simulink model "ATRIAS_anim_static_floor"  (R2014b)
settings: Solver=ode45  StartTime=0.0  StopTime=sim_t  FixedStep=1e-3  RelTol=1e-3  AbsTol=1e-4
undefined symbols (not defined in the file): base_color_d, boom_color_d, d_com, fblink_color_d, floor_color_d, floor_tile_width, floor_zero_height, g, hshaft_color_d, l_seg, lowerleg_12, lowerleg_color_d, m_boom, m_fblink, m_hshaft, m_lowerleg, m_output_gear, m_rotor, m_shin, m_thigh, m_torso, m_total, m_virtual_gear, m_yshaft, r_hip_gearhead, r_hip_shaft, r_rotor, r_virtual_gear, shin_12, shin_color_d, shin_initial_l, shin_initial_r, thigh_color_d, thigh_initial_l, thigh_initial_r, tile_color, tile_cross_section, tile_delta, tile_scale_visual, torso_color_d, X, Y, yshaft_color_d, Z
libraries: sm_lib x186, nesl_utility x85
(part 3 of 5)

== system ATRIAS_anim_static_floor/ATRIAS Mechanics Layer/ATRIAS Mechanical System Layer/L Hip Shaft/Frame Data ==
  Mux : Mux  Inputs=3
  PS-Simulink Converter{,1..3} (4 alike) : nesl_utility/PS-Simulink Converter  PhysicalDomain=network_engine_domain  SubClassName=ps_output  LeftPortType=input  RightPortType=output  PseudoPeriodic=off  Frequencies=[]  Unit=1  AffineConversion=off
  Transform Sensor : sm_lib/Frames and Transforms/Transform Sensor  MeasurementFrame=World  SenseAngle=off  SenseAxis=off  SenseAngle1=off  SenseAngle2=off  SenseAngle3=off  SenseQ=on  SenseR=off  SenseOmegaX=off  SenseOmegaY=off  SenseOmegaZ=off  SenseOmega1=off  SenseOmega2=off  SenseOmega3=off  SenseQDot=off  SenseRDot=off  SenseAlphaX=off  SenseAlphaY=off  SenseAlphaZ=off  SenseAlpha1=off  SenseAlpha2=off  SenseAlpha3=off  SenseQDDot=off  SenseRDDot=off  SenseX=on  SenseY=on  SenseZ=on  SenseRad=off  SenseAzim=off  SenseDist=off  SenseInc=off  SenseXDot=off  SenseYDot=off  SenseZDot=off  SenseRadDot=off  SenseAzimDot=off  SenseDistDot=off  SenseIncDot=off  SenseXDDot=off  SenseYDDot=off  SenseZDDot=off  SenseRadDDot=off  SenseAzimDDot=off  SenseDistDDot=off  SenseIncDDot=off  BlockFunction=simmechanics.library.frames_transforms.transform_sensor
  World Frame : sm_lib/Frames and Transforms/World Frame  BlockFunction=simmechanics.library.frames_transforms.world_frame
  Frame : PMIOPort  Port=1  Side=Left
  tag scope: LQHipShaft=global, LxyzHipShaft=global
  wires:
  PS-Simulink Converter/1 -> [LQHipShaft]
  PS-Simulink Converter1/1 -> Mux/1
  PS-Simulink Converter2/1 -> Mux/2
  PS-Simulink Converter3/1 -> Mux/3
  Mux/1 -> [LxyzHipShaft]
  connections:
  Transform Sensor/RConn1 -- Frame/RConn1
  Transform Sensor/LConn1 -- World Frame/RConn1
  Transform Sensor/RConn2 -- PS-Simulink Converter/LConn1
  Transform Sensor/RConn5 -- PS-Simulink Converter3/LConn1
  Transform Sensor/RConn3 -- PS-Simulink Converter1/LConn1
  Transform Sensor/RConn4 -- PS-Simulink Converter2/LConn1

== system ATRIAS_anim_static_floor/ATRIAS Mechanics Layer/ATRIAS Mechanical System Layer/L Leg/Angle Range Map1 ==
  "[0,2*pi]" : Inport
  Constant1 : Constant  Value=pi
  Constant2 : Constant  Value=pi
  Sum1 : Sum  Inputs=-+|
  Sum2 : Sum  Inputs=|+-
  Switch1 : Switch  ZeroCross=off
  "[-pi,pi]" : Outport
  wires:
  "[0,2*pi]"/1 -> Switch1/3, Sum1/2, Sum2/1
  Switch1/1 -> "[-pi,pi]"/1
  Constant2/1 -> Sum2/2
  Sum2/1 -> Switch1/2
  Sum1/1 -> Switch1/1
  Constant1/1 -> Sum1/1

== system ATRIAS_anim_static_floor/ATRIAS Mechanics Layer/ATRIAS Mechanical System Layer/L Leg/Angle Range Map2 ==
  "[0,2*pi]" : Inport
  Constant1 : Constant  Value=pi
  Constant2 : Constant  Value=pi
  Sum1 : Sum  Inputs=-+|
  Sum2 : Sum  Inputs=|+-
  Switch1 : Switch  ZeroCross=off
  "[-pi,pi]" : Outport
  wires:
  "[0,2*pi]"/1 -> Switch1/3, Sum1/2, Sum2/1
  Switch1/1 -> "[-pi,pi]"/1
  Constant2/1 -> Sum2/2
  Sum2/1 -> Switch1/2
  Sum1/1 -> Switch1/1
  Constant1/1 -> Sum1/1

== system ATRIAS_anim_static_floor/ATRIAS Mechanics Layer/ATRIAS Mechanical System Layer/L Leg/Four Bar Link ==
  CS1 to CS2 : sm_lib/Frames and Transforms/Rigid Transform  TranslationMethod=Cartesian  TranslationLengthUnit=m  TranslationStandardAxis=+Z  TranslationStandardOffset=0  TranslationCartesianOffset=[0 -l_seg 0]  TranslationROffset=0  TranslationROffsetUnits=m  TranslationZOffset=0  TranslationZOffsetUnits=m  TranslationThetaOffset=0  TranslationThetaOffsetUnits=deg  RotationMethod=None  RotationAngleUnits=deg  RotationStandardAxis=+Z  RotationAngle=0  RotationArbitraryAxis=[0 0 1]  FollAlignAxisA=+X  BaseAlignAxisA=+Y  FollAlignAxisB=+Y  BaseAlignAxisB=+Z  RotationMatrix=[1 0 0; 0 1 0; 0 0 1]  BlockFunction=simmechanics.library.frames_transforms.rigid_transform
  Frame Data : Subsystem
  Solid : sm_lib/Body Elements/Solid  InertiaType=Custom  Mass=m_fblink  MassUnits=kg  CenterOfMass=com_fblink  CenterOfMassUnits=m  MomentsOfInertia=i_fblink_moments  MomentsOfInertiaUnits=kg*m^2  ProductsOfInertia=i_fblink_products  ProductsOfInertiaUnits=kg*m^2  DensityBased=on  Density=1000  DensityUnits=kg/(m^3)  GraphicType=FromGeometry  MarkerShape=Sphere  MarkerSize=10  MarkerSizeUnits=m  GraphicVisPropType=AdvancedVisualProperties  GraphicDiffuseColor=fblink_color_d  GraphicSpecularColor=[0.5 0.5 0.5 1.0]  GraphicAmbientColor=[fblink_color_d*0.5 1.0]  GraphicEmissiveColor=[0.0 0.0 0.0 1.0]  GraphicShininess=128  GraphicOpacity=1.0  GeometryShape=FromFile  RectangleSize=[1 1]  RectangleSizeUnits=m  BrickDimensions=[0.1 l_seg 0.1]  BrickDimensionUnits=m  CylinderRadius=l_rad  CylinderRadiusUnits=m  CylinderLength=l_seg  CylinderLengthUnits=m  SphereRadius=1  SphereRadiusUnits=m  EllipsoidRadii=[1 1 1]  EllipsoidRadiiUnits=m  ExtrusionCrossSection=[1 1; -1 1; -1 -1; 1 -1]  ExtrusionCrossSectionUnits=m  ExtrusionLength=1  ExtrusionLengthUnits=m  PolygonNumSides=3  PolygonOuterRadius=1  PolygonOuterRadiusUnits=m  ExtGeomFileType=STL  ExtGeomFileName=../0_images/models/four_bar_link.stl  ExtGeomFileUnits=m  RevolutionCrossSection=[1 1; 1 -1; 2 -1; 2 1]  RevolutionCrossSectionUnits=m  RevolutionExtent=Full  RevolutionAngle=180  RevolutionAngleUnits=deg  BlockFunction=simmechanics.library.body_elements.solid
  CS1 : PMIOPort  Port=1  Side=Left
  CS2 : PMIOPort  Port=2  Side=Right
  connections:
  CS2/RConn1 -- CS1 to CS2/RConn1
  Solid/RConn1 -- CS1/RConn1 -- Frame Data/LConn1 -- CS1 to CS2/LConn1

== system ATRIAS_anim_static_floor/ATRIAS Mechanics Layer/ATRIAS Mechanical System Layer/L Leg/Lower Leg ==
  CS1 to CS2 : sm_lib/Frames and Transforms/Rigid Transform  TranslationMethod=Cartesian  TranslationLengthUnit=m  TranslationStandardAxis=+Z  TranslationStandardOffset=0  TranslationCartesianOffset=[0 -lowerleg_12 0]  TranslationROffset=0  TranslationROffsetUnits=m  TranslationZOffset=0  TranslationZOffsetUnits=m  TranslationThetaOffset=0  TranslationThetaOffsetUnits=deg  RotationMethod=None  RotationAngleUnits=deg  RotationStandardAxis=+Z  RotationAngle=0  RotationArbitraryAxis=[0 0 1]  FollAlignAxisA=+X  BaseAlignAxisA=+Y  FollAlignAxisB=+Y  BaseAlignAxisB=+Z  RotationMatrix=[1 0 0; 0 1 0; 0 0 1]  BlockFunction=simmechanics.library.frames_transforms.rigid_transform
  CS1 to CS3 : sm_lib/Frames and Transforms/Rigid Transform  TranslationMethod=Cartesian  TranslationLengthUnit=m  TranslationStandardAxis=+Z  TranslationStandardOffset=0  TranslationCartesianOffset=[0 -l_seg 0]  TranslationROffset=0  TranslationROffsetUnits=m  TranslationZOffset=0  TranslationZOffsetUnits=m  TranslationThetaOffset=0  TranslationThetaOffsetUnits=deg  RotationMethod=None  RotationAngleUnits=deg  RotationStandardAxis=+Z  RotationAngle=0  RotationArbitraryAxis=[0 0 1]  FollAlignAxisA=+X  BaseAlignAxisA=+Y  FollAlignAxisB=+Y  BaseAlignAxisB=+Z  RotationMatrix=[1 0 0; 0 1 0; 0 0 1]  BlockFunction=simmechanics.library.frames_transforms.rigid_transform
  Frame Data : Subsystem
  Solid : sm_lib/Body Elements/Solid  InertiaType=Custom  Mass=m_lowerleg  MassUnits=kg  CenterOfMass=com_lowerleg  CenterOfMassUnits=m  MomentsOfInertia=i_lowerleg_moments  MomentsOfInertiaUnits=kg*m^2  ProductsOfInertia=i_lowerleg_products  ProductsOfInertiaUnits=kg*m^2  DensityBased=on  Density=1000  DensityUnits=kg/(m^3)  GraphicType=FromGeometry  MarkerShape=Sphere  MarkerSize=10  MarkerSizeUnits=m  GraphicVisPropType=AdvancedVisualProperties  GraphicDiffuseColor=lowerleg_color_d  GraphicSpecularColor=[0.5 0.5 0.5 1.0]  GraphicAmbientColor=[lowerleg_color_d*0.5 1.0]  GraphicEmissiveColor=[0.0 0.0 0.0 1.0]  GraphicShininess=128  GraphicOpacity=1.0  GeometryShape=FromFile  RectangleSize=[1 1]  RectangleSizeUnits=m  BrickDimensions=[0.1 l_seg 0.1]  BrickDimensionUnits=m  CylinderRadius=l_rad  CylinderRadiusUnits=m  CylinderLength=l_seg  CylinderLengthUnits=m  SphereRadius=1  SphereRadiusUnits=m  EllipsoidRadii=[1 1 1]  EllipsoidRadiiUnits=m  ExtrusionCrossSection=[1 1; -1 1; -1 -1; 1 -1]  ExtrusionCrossSectionUnits=m  ExtrusionLength=1  ExtrusionLengthUnits=m  PolygonNumSides=3  PolygonOuterRadius=1  PolygonOuterRadiusUnits=m  ExtGeomFileType=STL  ExtGeomFileName=../0_images/models/lower_leg.STL  ExtGeomFileUnits=m  RevolutionCrossSection=[1 1; 1 -1; 2 -1; 2 1]  RevolutionCrossSectionUnits=m  RevolutionExtent=Full  RevolutionAngle=180  RevolutionAngleUnits=deg  BlockFunction=simmechanics.library.body_elements.solid
  CS1 : PMIOPort  Port=1  Side=Left
  CS2 : PMIOPort  Port=2  Side=Right
  CS3 : PMIOPort  Port=3  Side=Right
  connections:
  CS3/RConn1 -- CS1 to CS3/RConn1
  Frame Data/LConn1 -- CS1 to CS3/LConn1 -- CS1 to CS2/LConn1 -- Solid/RConn1 -- CS1/RConn1
  CS2/RConn1 -- CS1 to CS2/RConn1

== system ATRIAS_anim_static_floor/ATRIAS Mechanics Layer/ATRIAS Mechanical System Layer/L Leg/Shin ==
  CS1 to CS2 : sm_lib/Frames and Transforms/Rigid Transform  TranslationMethod=Cartesian  TranslationLengthUnit=m  TranslationStandardAxis=+Z  TranslationStandardOffset=0  TranslationCartesianOffset=[0 -shin_12 0]  TranslationROffset=0  TranslationROffsetUnits=m  TranslationZOffset=0  TranslationZOffsetUnits=m  TranslationThetaOffset=0  TranslationThetaOffsetUnits=deg  RotationMethod=None  RotationAngleUnits=deg  RotationStandardAxis=+Z  RotationAngle=0  RotationArbitraryAxis=[0 0 1]  FollAlignAxisA=+X  BaseAlignAxisA=+Y  FollAlignAxisB=+Y  BaseAlignAxisB=+Z  RotationMatrix=[1 0 0; 0 1 0; 0 0 1]  BlockFunction=simmechanics.library.frames_transforms.rigid_transform
  Frame Data : Subsystem
  Solid : sm_lib/Body Elements/Solid  InertiaType=Custom  Mass=m_shin  MassUnits=kg  CenterOfMass=com_shin  CenterOfMassUnits=m  MomentsOfInertia=i_shin_moments  MomentsOfInertiaUnits=kg*m^2  ProductsOfInertia=i_shin_products  ProductsOfInertiaUnits=kg*m^2  DensityBased=on  Density=1000  DensityUnits=kg/(m^3)  GraphicType=FromGeometry  MarkerShape=Sphere  MarkerSize=10  MarkerSizeUnits=m  GraphicVisPropType=AdvancedVisualProperties  GraphicDiffuseColor=shin_color_d  GraphicSpecularColor=[0.5 0.5 0.5 1.0]  GraphicAmbientColor=[shin_color_d*0.5 1.0]  GraphicEmissiveColor=[0.0 0.0 0.0 1.0]  GraphicShininess=128  GraphicOpacity=1.0  GeometryShape=FromFile  RectangleSize=[1 1]  RectangleSizeUnits=m  BrickDimensions=[1 1 1]  BrickDimensionUnits=m  CylinderRadius=l_rad  CylinderRadiusUnits=m  CylinderLength=l_seg  CylinderLengthUnits=m  SphereRadius=1  SphereRadiusUnits=m  EllipsoidRadii=[1 1 1]  EllipsoidRadiiUnits=m  ExtrusionCrossSection=[1 1; -1 1; -1 -1; 1 -1]  ExtrusionCrossSectionUnits=m  ExtrusionLength=1  ExtrusionLengthUnits=m  PolygonNumSides=3  PolygonOuterRadius=1  PolygonOuterRadiusUnits=m  ExtGeomFileType=STL  ExtGeomFileName=../0_images/models/shin.STL  ExtGeomFileUnits=m  RevolutionCrossSection=[1 1; 1 -1; 2 -1; 2 1]  RevolutionCrossSectionUnits=m  RevolutionExtent=Full  RevolutionAngle=180  RevolutionAngleUnits=deg  BlockFunction=simmechanics.library.body_elements.solid
  CS1 : PMIOPort  Port=1  Side=Left
  CS2 : PMIOPort  Port=2  Side=Right
  connections:
  CS1 to CS2/LConn1 -- CS1/RConn1 -- Frame Data/LConn1 -- Solid/RConn1
  CS2/RConn1 -- CS1 to CS2/RConn1

== system ATRIAS_anim_static_floor/ATRIAS Mechanics Layer/ATRIAS Mechanical System Layer/L Leg/Shin SEA ==
  note: Shin SEA Mechanics
  Shin Gear [rad] : Inport
  Initial Gear Angle1 : Constant  Value=shin_initial_l
  Rotor and Gearing : Subsystem
  Sum1 : Sum  Inputs=-+|
  Terminator : Terminator
  Terminator1 : Terminator
  Rotor Joint Conn : PMIOPort  Port=1  Side=Left
  wires:
  Rotor and Gearing/2(Gearhead Velocity [rad/s]) -> Terminator/1
  Sum1/1 -> Rotor and Gearing/1(Shin Gear pos [rad])
  Shin Gear [rad]/1 -> Sum1/2
  Initial Gear Angle1/1 -> Sum1/1
  Rotor and Gearing/1(Gearhead Position [rad]) -> Terminator1/1
  connections:
  Rotor and Gearing/LConn1 -- Rotor Joint Conn/RConn1

== system ATRIAS_anim_static_floor/ATRIAS Mechanics Layer/ATRIAS Mechanical System Layer/L Leg/Thigh ==
  CS1 to CS2 : sm_lib/Frames and Transforms/Rigid Transform  TranslationMethod=Cartesian  TranslationLengthUnit=m  TranslationStandardAxis=+Z  TranslationStandardOffset=0  TranslationCartesianOffset=[0 -l_seg 0]  TranslationROffset=0  TranslationROffsetUnits=m  TranslationZOffset=0  TranslationZOffsetUnits=m  TranslationThetaOffset=0  TranslationThetaOffsetUnits=deg  RotationMethod=None  RotationAngleUnits=deg  RotationStandardAxis=+Z  RotationAngle=0  RotationArbitraryAxis=[0 0 1]  FollAlignAxisA=+X  BaseAlignAxisA=+Y  FollAlignAxisB=+Y  BaseAlignAxisB=+Z  RotationMatrix=[1 0 0; 0 1 0; 0 0 1]  BlockFunction=simmechanics.library.frames_transforms.rigid_transform
  Frame Data : Subsystem
  Solid : sm_lib/Body Elements/Solid  InertiaType=Custom  Mass=m_thigh  MassUnits=kg  CenterOfMass=com_thigh  CenterOfMassUnits=m  MomentsOfInertia=i_thigh_moments  MomentsOfInertiaUnits=kg*m^2  ProductsOfInertia=i_thigh_products  ProductsOfInertiaUnits=kg*m^2  DensityBased=on  Density=1000  DensityUnits=kg/(m^3)  GraphicType=FromGeometry  MarkerShape=Sphere  MarkerSize=10  MarkerSizeUnits=m  GraphicVisPropType=AdvancedVisualProperties  GraphicDiffuseColor=thigh_color_d  GraphicSpecularColor=[0.5 0.5 0.5 1.0]  GraphicAmbientColor=[thigh_color_d*0.5 1.0]  GraphicEmissiveColor=[0.0 0.0 0.0 1.0]  GraphicShininess=128  GraphicOpacity=1.0  GeometryShape=FromFile  RectangleSize=[1 1]  RectangleSizeUnits=m  BrickDimensions=[1 1 1]  BrickDimensionUnits=m  CylinderRadius=l_rad  CylinderRadiusUnits=m  CylinderLength=l_seg  CylinderLengthUnits=m  SphereRadius=1  SphereRadiusUnits=m  EllipsoidRadii=[1 1 1]  EllipsoidRadiiUnits=m  ExtrusionCrossSection=[1 1; -1 1; -1 -1; 1 -1]  ExtrusionCrossSectionUnits=m  ExtrusionLength=1  ExtrusionLengthUnits=m  PolygonNumSides=3  PolygonOuterRadius=1  PolygonOuterRadiusUnits=m  ExtGeomFileType=STL  ExtGeomFileName=../0_images/models/thigh.STL  ExtGeomFileUnits=m  RevolutionCrossSection=[1 1; 1 -1; 2 -1; 2 1]  RevolutionCrossSectionUnits=m  RevolutionExtent=Full  RevolutionAngle=180  RevolutionAngleUnits=deg  BlockFunction=simmechanics.library.body_elements.solid
  CS1 : PMIOPort  Port=1  Side=Left
  CS2 : PMIOPort  Port=2  Side=Right
  connections:
  CS2/RConn1 -- CS1 to CS2/RConn1
  CS1 to CS2/LConn1 -- Solid/RConn1 -- Frame Data/LConn1 -- CS1/RConn1

== system ATRIAS_anim_static_floor/ATRIAS Mechanics Layer/ATRIAS Mechanical System Layer/L Leg/Thigh SEA ==
  note: Thigh SEA Mechanics
  Thigh Gear [rad] : Inport
  Initial Gear Angle1 : Constant  Value=thigh_initial_l
  Rotor and Gearing : Subsystem
  Sum1 : Sum  Inputs=-+|
  Terminator : Terminator
  Terminator1 : Terminator
  Rotor Joint Conn : PMIOPort  Port=1  Side=Left
  wires:
  Rotor and Gearing/2(Gearhead Velocity [rad/s]) -> Terminator/1
  Sum1/1 -> Rotor and Gearing/1(Thigh Gear pos [rad])
  Initial Gear Angle1/1 -> Sum1/1
  Thigh Gear [rad]/1 -> Sum1/2
  Rotor and Gearing/1(Gearhead Position [rad]) -> Terminator1/1
  connections:
  Rotor and Gearing/LConn1 -- Rotor Joint Conn/RConn1

== system ATRIAS_anim_static_floor/ATRIAS Mechanics Layer/ATRIAS Mechanical System Layer/R Hip Shaft/Frame Data ==
  Mux : Mux  Inputs=3
  PS-Simulink Converter{,1..3} (4 alike) : nesl_utility/PS-Simulink Converter  PhysicalDomain=network_engine_domain  SubClassName=ps_output  LeftPortType=input  RightPortType=output  PseudoPeriodic=off  Frequencies=[]  Unit=1  AffineConversion=off
  Transform Sensor : sm_lib/Frames and Transforms/Transform Sensor  MeasurementFrame=World  SenseAngle=off  SenseAxis=off  SenseAngle1=off  SenseAngle2=off  SenseAngle3=off  SenseQ=on  SenseR=off  SenseOmegaX=off  SenseOmegaY=off  SenseOmegaZ=off  SenseOmega1=off  SenseOmega2=off  SenseOmega3=off  SenseQDot=off  SenseRDot=off  SenseAlphaX=off  SenseAlphaY=off  SenseAlphaZ=off  SenseAlpha1=off  SenseAlpha2=off  SenseAlpha3=off  SenseQDDot=off  SenseRDDot=off  SenseX=on  SenseY=on  SenseZ=on  SenseRad=off  SenseAzim=off  SenseDist=off  SenseInc=off  SenseXDot=off  SenseYDot=off  SenseZDot=off  SenseRadDot=off  SenseAzimDot=off  SenseDistDot=off  SenseIncDot=off  SenseXDDot=off  SenseYDDot=off  SenseZDDot=off  SenseRadDDot=off  SenseAzimDDot=off  SenseDistDDot=off  SenseIncDDot=off  BlockFunction=simmechanics.library.frames_transforms.transform_sensor
  World Frame : sm_lib/Frames and Transforms/World Frame  BlockFunction=simmechanics.library.frames_transforms.world_frame
  Frame : PMIOPort  Port=1  Side=Left
  tag scope: RQHipShaft=global, RxyzHipShaft=global
  wires:
  PS-Simulink Converter/1 -> [RQHipShaft]
  PS-Simulink Converter1/1 -> Mux/1
  PS-Simulink Converter2/1 -> Mux/2
  PS-Simulink Converter3/1 -> Mux/3
  Mux/1 -> [RxyzHipShaft]
  connections:
  Transform Sensor/RConn1 -- Frame/RConn1
  Transform Sensor/LConn1 -- World Frame/RConn1
  Transform Sensor/RConn3 -- PS-Simulink Converter1/LConn1
  Transform Sensor/RConn5 -- PS-Simulink Converter3/LConn1
  Transform Sensor/RConn4 -- PS-Simulink Converter2/LConn1
  Transform Sensor/RConn2 -- PS-Simulink Converter/LConn1

== system ATRIAS_anim_static_floor/ATRIAS Mechanics Layer/ATRIAS Mechanical System Layer/R Leg/Angle Range Map1 ==
  "[0,2*pi]" : Inport
  Constant1 : Constant  Value=pi
  Constant2 : Constant  Value=pi
  Sum1 : Sum  Inputs=-+|
  Sum2 : Sum  Inputs=|+-
  Switch1 : Switch  ZeroCross=off
  "[-pi,pi]" : Outport
  wires:
  "[0,2*pi]"/1 -> Switch1/3, Sum1/2, Sum2/1
  Switch1/1 -> "[-pi,pi]"/1
  Constant2/1 -> Sum2/2
  Sum2/1 -> Switch1/2
  Sum1/1 -> Switch1/1
  Constant1/1 -> Sum1/1

== system ATRIAS_anim_static_floor/ATRIAS Mechanics Layer/ATRIAS Mechanical System Layer/R Leg/Angle Range Map2 ==
  "[0,2*pi]" : Inport
  Constant1 : Constant  Value=pi
  Constant2 : Constant  Value=pi
  Sum1 : Sum  Inputs=-+|
  Sum2 : Sum  Inputs=|+-
  Switch1 : Switch  ZeroCross=off
  "[-pi,pi]" : Outport
  wires:
  "[0,2*pi]"/1 -> Switch1/3, Sum1/2, Sum2/1
  Switch1/1 -> "[-pi,pi]"/1
  Constant2/1 -> Sum2/2
  Sum2/1 -> Switch1/2
  Sum1/1 -> Switch1/1
  Constant1/1 -> Sum1/1

== system ATRIAS_anim_static_floor/ATRIAS Mechanics Layer/ATRIAS Mechanical System Layer/R Leg/Four Bar Link ==
  CS1 to CS2 : sm_lib/Frames and Transforms/Rigid Transform  TranslationMethod=Cartesian  TranslationLengthUnit=m  TranslationStandardAxis=+Z  TranslationStandardOffset=0  TranslationCartesianOffset=[0 -l_seg 0]  TranslationROffset=0  TranslationROffsetUnits=m  TranslationZOffset=0  TranslationZOffsetUnits=m  TranslationThetaOffset=0  TranslationThetaOffsetUnits=deg  RotationMethod=None  RotationAngleUnits=deg  RotationStandardAxis=+Z  RotationAngle=0  RotationArbitraryAxis=[0 0 1]  FollAlignAxisA=+X  BaseAlignAxisA=+Y  FollAlignAxisB=+Y  BaseAlignAxisB=+Z  RotationMatrix=[1 0 0; 0 1 0; 0 0 1]  BlockFunction=simmechanics.library.frames_transforms.rigid_transform
  Frame Data : Subsystem
  Solid : sm_lib/Body Elements/Solid  InertiaType=Custom  Mass=m_fblink  MassUnits=kg  CenterOfMass=com_fblink  CenterOfMassUnits=m  MomentsOfInertia=i_fblink_moments  MomentsOfInertiaUnits=kg*m^2  ProductsOfInertia=i_fblink_products  ProductsOfInertiaUnits=kg*m^2  DensityBased=on  Density=1000  DensityUnits=kg/(m^3)  GraphicType=FromGeometry  MarkerShape=Sphere  MarkerSize=10  MarkerSizeUnits=m  GraphicVisPropType=AdvancedVisualProperties  GraphicDiffuseColor=fblink_color_d  GraphicSpecularColor=[0.5 0.5 0.5 1.0]  GraphicAmbientColor=[fblink_color_d*0.5 1.0]  GraphicEmissiveColor=[0.0 0.0 0.0 1.0]  GraphicShininess=128  GraphicOpacity=1.0  GeometryShape=FromFile  RectangleSize=[1 1]  RectangleSizeUnits=m  BrickDimensions=[0.1 l_seg 0.1]  BrickDimensionUnits=m  CylinderRadius=l_rad  CylinderRadiusUnits=m  CylinderLength=l_seg  CylinderLengthUnits=m  SphereRadius=1  SphereRadiusUnits=m  EllipsoidRadii=[1 1 1]  EllipsoidRadiiUnits=m  ExtrusionCrossSection=[1 1; -1 1; -1 -1; 1 -1]  ExtrusionCrossSectionUnits=m  ExtrusionLength=1  ExtrusionLengthUnits=m  PolygonNumSides=3  PolygonOuterRadius=1  PolygonOuterRadiusUnits=m  ExtGeomFileType=STL  ExtGeomFileName=../0_images/models/four_bar_link.stl  ExtGeomFileUnits=m  RevolutionCrossSection=[1 1; 1 -1; 2 -1; 2 1]  RevolutionCrossSectionUnits=m  RevolutionExtent=Full  RevolutionAngle=180  RevolutionAngleUnits=deg  BlockFunction=simmechanics.library.body_elements.solid
  CS1 : PMIOPort  Port=1  Side=Left
  CS2 : PMIOPort  Port=2  Side=Right
  connections:
  CS2/RConn1 -- CS1 to CS2/RConn1
  Solid/RConn1 -- CS1/RConn1 -- Frame Data/LConn1 -- CS1 to CS2/LConn1

== system ATRIAS_anim_static_floor/ATRIAS Mechanics Layer/ATRIAS Mechanical System Layer/R Leg/Lower Leg ==
  CS1 to CS2 : sm_lib/Frames and Transforms/Rigid Transform  TranslationMethod=Cartesian  TranslationLengthUnit=m  TranslationStandardAxis=+Z  TranslationStandardOffset=0  TranslationCartesianOffset=[0 -lowerleg_12 0]  TranslationROffset=0  TranslationROffsetUnits=m  TranslationZOffset=0  TranslationZOffsetUnits=m  TranslationThetaOffset=0  TranslationThetaOffsetUnits=deg  RotationMethod=None  RotationAngleUnits=deg  RotationStandardAxis=+Z  RotationAngle=0  RotationArbitraryAxis=[0 0 1]  FollAlignAxisA=+X  BaseAlignAxisA=+Y  FollAlignAxisB=+Y  BaseAlignAxisB=+Z  RotationMatrix=[1 0 0; 0 1 0; 0 0 1]  BlockFunction=simmechanics.library.frames_transforms.rigid_transform
  CS1 to CS3 : sm_lib/Frames and Transforms/Rigid Transform  TranslationMethod=Cartesian  TranslationLengthUnit=m  TranslationStandardAxis=+Z  TranslationStandardOffset=0  TranslationCartesianOffset=[0 -l_seg 0]  TranslationROffset=0  TranslationROffsetUnits=m  TranslationZOffset=0  TranslationZOffsetUnits=m  TranslationThetaOffset=0  TranslationThetaOffsetUnits=deg  RotationMethod=None  RotationAngleUnits=deg  RotationStandardAxis=+Z  RotationAngle=0  RotationArbitraryAxis=[0 0 1]  FollAlignAxisA=+X  BaseAlignAxisA=+Y  FollAlignAxisB=+Y  BaseAlignAxisB=+Z  RotationMatrix=[1 0 0; 0 1 0; 0 0 1]  BlockFunction=simmechanics.library.frames_transforms.rigid_transform
  Frame Data : Subsystem
  Solid : sm_lib/Body Elements/Solid  InertiaType=Custom  Mass=m_lowerleg  MassUnits=kg  CenterOfMass=com_lowerleg  CenterOfMassUnits=m  MomentsOfInertia=i_lowerleg_moments  MomentsOfInertiaUnits=kg*m^2  ProductsOfInertia=i_lowerleg_products  ProductsOfInertiaUnits=kg*m^2  DensityBased=on  Density=1000  DensityUnits=kg/(m^3)  GraphicType=FromGeometry  MarkerShape=Sphere  MarkerSize=10  MarkerSizeUnits=m  GraphicVisPropType=AdvancedVisualProperties  GraphicDiffuseColor=lowerleg_color_d  GraphicSpecularColor=[0.5 0.5 0.5 1.0]  GraphicAmbientColor=[lowerleg_color_d*0.5 1.0]  GraphicEmissiveColor=[0.0 0.0 0.0 1.0]  GraphicShininess=128  GraphicOpacity=1.0  GeometryShape=FromFile  RectangleSize=[1 1]  RectangleSizeUnits=m  BrickDimensions=[0.1 l_seg 0.1]  BrickDimensionUnits=m  CylinderRadius=l_rad  CylinderRadiusUnits=m  CylinderLength=l_seg  CylinderLengthUnits=m  SphereRadius=1  SphereRadiusUnits=m  EllipsoidRadii=[1 1 1]  EllipsoidRadiiUnits=m  ExtrusionCrossSection=[1 1; -1 1; -1 -1; 1 -1]  ExtrusionCrossSectionUnits=m  ExtrusionLength=1  ExtrusionLengthUnits=m  PolygonNumSides=3  PolygonOuterRadius=1  PolygonOuterRadiusUnits=m  ExtGeomFileType=STL  ExtGeomFileName=../0_images/models/lower_leg.STL  ExtGeomFileUnits=m  RevolutionCrossSection=[1 1; 1 -1; 2 -1; 2 1]  RevolutionCrossSectionUnits=m  RevolutionExtent=Full  RevolutionAngle=180  RevolutionAngleUnits=deg  BlockFunction=simmechanics.library.body_elements.solid
  CS1 : PMIOPort  Port=1  Side=Left
  CS2 : PMIOPort  Port=2  Side=Right
  CS3 : PMIOPort  Port=3  Side=Right
  connections:
  CS3/RConn1 -- CS1 to CS3/RConn1
  CS1 to CS3/LConn1 -- CS1 to CS2/LConn1 -- Solid/RConn1 -- Frame Data/LConn1 -- CS1/RConn1
  CS2/RConn1 -- CS1 to CS2/RConn1

== system ATRIAS_anim_static_floor/ATRIAS Mechanics Layer/ATRIAS Mechanical System Layer/R Leg/Shin ==
  CS1 to CS2 : sm_lib/Frames and Transforms/Rigid Transform  TranslationMethod=Cartesian  TranslationLengthUnit=m  TranslationStandardAxis=+Z  TranslationStandardOffset=0  TranslationCartesianOffset=[0 -shin_12 0]  TranslationROffset=0  TranslationROffsetUnits=m  TranslationZOffset=0  TranslationZOffsetUnits=m  TranslationThetaOffset=0  TranslationThetaOffsetUnits=deg  RotationMethod=None  RotationAngleUnits=deg  RotationStandardAxis=+Z  RotationAngle=0  RotationArbitraryAxis=[0 0 1]  FollAlignAxisA=+X  BaseAlignAxisA=+Y  FollAlignAxisB=+Y  BaseAlignAxisB=+Z  RotationMatrix=[1 0 0; 0 1 0; 0 0 1]  BlockFunction=simmechanics.library.frames_transforms.rigid_transform
  Frame Data : Subsystem
  Solid : sm_lib/Body Elements/Solid  InertiaType=Custom  Mass=m_shin  MassUnits=kg  CenterOfMass=com_shin  CenterOfMassUnits=m  MomentsOfInertia=i_shin_moments  MomentsOfInertiaUnits=kg*m^2  ProductsOfInertia=i_shin_products  ProductsOfInertiaUnits=kg*m^2  DensityBased=on  Density=1000  DensityUnits=kg/(m^3)  GraphicType=FromGeometry  MarkerShape=Sphere  MarkerSize=10  MarkerSizeUnits=m  GraphicVisPropType=AdvancedVisualProperties  GraphicDiffuseColor=shin_color_d  GraphicSpecularColor=[0.5 0.5 0.5 1.0]  GraphicAmbientColor=[shin_color_d*0.5 1.0]  GraphicEmissiveColor=[0.0 0.0 0.0 1.0]  GraphicShininess=128  GraphicOpacity=1.0  GeometryShape=FromFile  RectangleSize=[1 1]  RectangleSizeUnits=m  BrickDimensions=[1 1 1]  BrickDimensionUnits=m  CylinderRadius=l_rad  CylinderRadiusUnits=m  CylinderLength=l_seg  CylinderLengthUnits=m  SphereRadius=1  SphereRadiusUnits=m  EllipsoidRadii=[1 1 1]  EllipsoidRadiiUnits=m  ExtrusionCrossSection=[1 1; -1 1; -1 -1; 1 -1]  ExtrusionCrossSectionUnits=m  ExtrusionLength=1  ExtrusionLengthUnits=m  PolygonNumSides=3  PolygonOuterRadius=1  PolygonOuterRadiusUnits=m  ExtGeomFileType=STL  ExtGeomFileName=../0_images/models/shin.STL  ExtGeomFileUnits=m  RevolutionCrossSection=[1 1; 1 -1; 2 -1; 2 1]  RevolutionCrossSectionUnits=m  RevolutionExtent=Full  RevolutionAngle=180  RevolutionAngleUnits=deg  BlockFunction=simmechanics.library.body_elements.solid
  CS1 : PMIOPort  Port=1  Side=Left
  CS2 : PMIOPort  Port=2  Side=Right
  connections:
  CS1 to CS2/LConn1 -- CS1/RConn1 -- Frame Data/LConn1 -- Solid/RConn1
  CS2/RConn1 -- CS1 to CS2/RConn1

== system ATRIAS_anim_static_floor/ATRIAS Mechanics Layer/ATRIAS Mechanical System Layer/R Leg/Shin SEA ==
  note: Shin SEA Mechanics
  Shin Gear Pos [rad] : Inport
  Initial Gear Angle1 : Constant  Value=shin_initial_r
  Rotor and Gearing : Subsystem
  Sum1 : Sum  Inputs=-+|
  Terminator : Terminator
  Terminator1 : Terminator
  Rotor Joint Conn : PMIOPort  Port=1  Side=Left
  wires:
  Sum1/1 -> Rotor and Gearing/1(Gear position [rad])
  Shin Gear Pos [rad]/1 -> Sum1/2
  Initial Gear Angle1/1 -> Sum1/1
  Rotor and Gearing/2(Gearhead Velocity [rad/s]) -> Terminator/1
  Rotor and Gearing/1(Gearhead Position [rad]) -> Terminator1/1
  connections:
  Rotor and Gearing/LConn1 -- Rotor Joint Conn/RConn1

== system ATRIAS_anim_static_floor/ATRIAS Mechanics Layer/ATRIAS Mechanical System Layer/R Leg/Thigh ==
  CS1 to CS2 : sm_lib/Frames and Transforms/Rigid Transform  TranslationMethod=Cartesian  TranslationLengthUnit=m  TranslationStandardAxis=+Z  TranslationStandardOffset=0  TranslationCartesianOffset=[0 -l_seg 0]  TranslationROffset=0  TranslationROffsetUnits=m  TranslationZOffset=0  TranslationZOffsetUnits=m  TranslationThetaOffset=0  TranslationThetaOffsetUnits=deg  RotationMethod=None  RotationAngleUnits=deg  RotationStandardAxis=+Z  RotationAngle=0  RotationArbitraryAxis=[0 0 1]  FollAlignAxisA=+X  BaseAlignAxisA=+Y  FollAlignAxisB=+Y  BaseAlignAxisB=+Z  RotationMatrix=[1 0 0; 0 1 0; 0 0 1]  BlockFunction=simmechanics.library.frames_transforms.rigid_transform
  Frame Data : Subsystem
  Solid : sm_lib/Body Elements/Solid  InertiaType=Custom  Mass=m_thigh  MassUnits=kg  CenterOfMass=com_thigh  CenterOfMassUnits=m  MomentsOfInertia=i_thigh_moments  MomentsOfInertiaUnits=kg*m^2  ProductsOfInertia=i_thigh_products  ProductsOfInertiaUnits=kg*m^2  DensityBased=on  Density=1000  DensityUnits=kg/(m^3)  GraphicType=FromGeometry  MarkerShape=Sphere  MarkerSize=10  MarkerSizeUnits=m  GraphicVisPropType=AdvancedVisualProperties  GraphicDiffuseColor=thigh_color_d  GraphicSpecularColor=[0.5 0.5 0.5 1.0]  GraphicAmbientColor=[thigh_color_d*0.5 1.0]  GraphicEmissiveColor=[0.0 0.0 0.0 1.0]  GraphicShininess=128  GraphicOpacity=1.0  GeometryShape=FromFile  RectangleSize=[1 1]  RectangleSizeUnits=m  BrickDimensions=[1 1 1]  BrickDimensionUnits=m  CylinderRadius=l_rad  CylinderRadiusUnits=m  CylinderLength=l_seg  CylinderLengthUnits=m  SphereRadius=1  SphereRadiusUnits=m  EllipsoidRadii=[1 1 1]  EllipsoidRadiiUnits=m  ExtrusionCrossSection=[1 1; -1 1; -1 -1; 1 -1]  ExtrusionCrossSectionUnits=m  ExtrusionLength=1  ExtrusionLengthUnits=m  PolygonNumSides=3  PolygonOuterRadius=1  PolygonOuterRadiusUnits=m  ExtGeomFileType=STL  ExtGeomFileName=../0_images/models/thigh.STL  ExtGeomFileUnits=m  RevolutionCrossSection=[1 1; 1 -1; 2 -1; 2 1]  RevolutionCrossSectionUnits=m  RevolutionExtent=Full  RevolutionAngle=180  RevolutionAngleUnits=deg  BlockFunction=simmechanics.library.body_elements.solid
  CS1 : PMIOPort  Port=1  Side=Left
  CS2 : PMIOPort  Port=2  Side=Right
  connections:
  CS2/RConn1 -- CS1 to CS2/RConn1
  CS1 to CS2/LConn1 -- Solid/RConn1 -- Frame Data/LConn1 -- CS1/RConn1

== system ATRIAS_anim_static_floor/ATRIAS Mechanics Layer/ATRIAS Mechanical System Layer/R Leg/Thigh SEA ==
  note: Thigh SEA Mechanics
  Thigh Gear [rad] : Inport
  Initial Gear Angle1 : Constant  Value=thigh_initial_r
  Rotor and Gearing : Subsystem
  Sum1 : Sum  Inputs=-+|
  Terminator : Terminator
  Terminator1 : Terminator
  Rotor Joint Conn : PMIOPort  Port=1  Side=Left
  wires:
  Sum1/1 -> Rotor and Gearing/1(Thigh Gear pos [rad])
  Initial Gear Angle1/1 -> Sum1/1
  Thigh Gear [rad]/1 -> Sum1/2
  Rotor and Gearing/2(Gearhead Velocity [rad/s]) -> Terminator/1
  Rotor and Gearing/1(Gearhead Position [rad]) -> Terminator1/1
  connections:
  Rotor and Gearing/LConn1 -- Rotor Joint Conn/RConn1

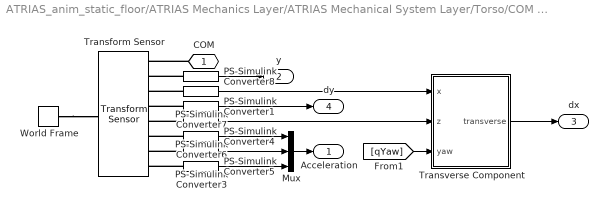
== system ATRIAS_anim_static_floor/ATRIAS Mechanics Layer/ATRIAS Mechanical System Layer/Torso/COM Sensor ==
  Mux : Mux  Inputs=3
  PS-Simulink Converter{1,3..8} (7 alike) : nesl_utility/PS-Simulink Converter  PhysicalDomain=network_engine_domain  SubClassName=ps_output  LeftPortType=input  RightPortType=output  PseudoPeriodic=off  Frequencies=[]  Unit=1  AffineConversion=off
  Transform Sensor : sm_lib/Frames and Transforms/Transform Sensor  MeasurementFrame=World  SenseAngle=off  SenseAxis=off  SenseAngle1=off  SenseAngle2=off  SenseAngle3=off  SenseQ=off  SenseR=off  SenseOmegaX=off  SenseOmegaY=off  SenseOmegaZ=off  SenseOmega1=off  SenseOmega2=off  SenseOmega3=off  SenseQDot=off  SenseRDot=off  SenseAlphaX=off  SenseAlphaY=off  SenseAlphaZ=off  SenseAlpha1=off  SenseAlpha2=off  SenseAlpha3=off  SenseQDDot=off  SenseRDDot=off  SenseX=off  SenseY=on  SenseZ=off  SenseRad=off  SenseAzim=off  SenseDist=off  SenseInc=off  SenseXDot=on  SenseYDot=on  SenseZDot=on  SenseRadDot=off  SenseAzimDot=off  SenseDistDot=off  SenseIncDot=off  SenseXDDot=on  SenseYDDot=on  SenseZDDot=on  SenseRadDDot=off  SenseAzimDDot=off  SenseDistDDot=off  SenseIncDDot=off  BlockFunction=simmechanics.library.frames_transforms.transform_sensor
  Transverse Component : Subsystem
  World Frame : sm_lib/Frames and Transforms/World Frame  BlockFunction=simmechanics.library.frames_transforms.world_frame
  COM : PMIOPort  Port=1  Side=Left
  Acceleration : Outport
  y : Outport  Port=2
  dx : Outport  Port=3
  dy : Outport  Port=4
  wires:
  PS-Simulink Converter5/1 -> Mux/3
  Mux/1 -> Acceleration/1
  PS-Simulink Converter8/1 -> y/1
  PS-Simulink Converter3/1 -> Mux/2
  PS-Simulink Converter4/1 -> Mux/1
  PS-Simulink Converter7/1 -> Transverse Component/1(x)
  Transverse Component/1(transverse) -> dx/1
  [qYaw] -> Transverse Component/3(yaw)
  PS-Simulink Converter1/1 -> dy/1
  PS-Simulink Converter6/1 -> Transverse Component/2(z)
  connections:
  COM/RConn1 -- Transform Sensor/RConn1
  World Frame/RConn1 -- Transform Sensor/LConn1
  PS-Simulink Converter5/LConn1 -- Transform Sensor/RConn8
  PS-Simulink Converter3/LConn1 -- Transform Sensor/RConn7
  PS-Simulink Converter4/LConn1 -- Transform Sensor/RConn6
  PS-Simulink Converter6/LConn1 -- Transform Sensor/RConn5
  PS-Simulink Converter7/LConn1 -- Transform Sensor/RConn3
  PS-Simulink Converter8/LConn1 -- Transform Sensor/RConn2
  PS-Simulink Converter1/LConn1 -- Transform Sensor/RConn4

== system ATRIAS_anim_static_floor/ATRIAS Mechanics Layer/ATRIAS Mechanical System Layer/Torso/Frame Data ==
  Mux : Mux  Inputs=3
  PS-Simulink Converter{,1..3} (4 alike) : nesl_utility/PS-Simulink Converter  PhysicalDomain=network_engine_domain  SubClassName=ps_output  LeftPortType=input  RightPortType=output  PseudoPeriodic=off  Frequencies=[]  Unit=1  AffineConversion=off
  Transform Sensor : sm_lib/Frames and Transforms/Transform Sensor  MeasurementFrame=World  SenseAngle=off  SenseAxis=off  SenseAngle1=off  SenseAngle2=off  SenseAngle3=off  SenseQ=on  SenseR=off  SenseOmegaX=off  SenseOmegaY=off  SenseOmegaZ=off  SenseOmega1=off  SenseOmega2=off  SenseOmega3=off  SenseQDot=off  SenseRDot=off  SenseAlphaX=off  SenseAlphaY=off  SenseAlphaZ=off  SenseAlpha1=off  SenseAlpha2=off  SenseAlpha3=off  SenseQDDot=off  SenseRDDot=off  SenseX=on  SenseY=on  SenseZ=on  SenseRad=off  SenseAzim=off  SenseDist=off  SenseInc=off  SenseXDot=off  SenseYDot=off  SenseZDot=off  SenseRadDot=off  SenseAzimDot=off  SenseDistDot=off  SenseIncDot=off  SenseXDDot=off  SenseYDDot=off  SenseZDDot=off  SenseRadDDot=off  SenseAzimDDot=off  SenseDistDDot=off  SenseIncDDot=off  BlockFunction=simmechanics.library.frames_transforms.transform_sensor
  World Frame : sm_lib/Frames and Transforms/World Frame  BlockFunction=simmechanics.library.frames_transforms.world_frame
  Frame : PMIOPort  Port=1  Side=Left
  tag scope: QTorso=global, xyzTorso=global
  wires:
  PS-Simulink Converter/1 -> [QTorso]
  PS-Simulink Converter1/1 -> Mux/1
  PS-Simulink Converter2/1 -> Mux/2
  PS-Simulink Converter3/1 -> Mux/3
  Mux/1 -> [xyzTorso]
  connections:
  Transform Sensor/RConn1 -- Frame/RConn1
  Transform Sensor/LConn1 -- World Frame/RConn1
  Transform Sensor/RConn5 -- PS-Simulink Converter3/LConn1
  Transform Sensor/RConn4 -- PS-Simulink Converter2/LConn1
  Transform Sensor/RConn3 -- PS-Simulink Converter1/LConn1
  Transform Sensor/RConn2 -- PS-Simulink Converter/LConn1

== system ATRIAS_anim_static_floor/ATRIAS Mechanics Layer/ATRIAS Mechanical System Layer/Yaw Shaft/Frame Data ==
  Mux : Mux  Inputs=3
  PS-Simulink Converter{,1..3} (4 alike) : nesl_utility/PS-Simulink Converter  PhysicalDomain=network_engine_domain  SubClassName=ps_output  LeftPortType=input  RightPortType=output  PseudoPeriodic=off  Frequencies=[]  Unit=1  AffineConversion=off
  Transform Sensor : sm_lib/Frames and Transforms/Transform Sensor  MeasurementFrame=World  SenseAngle=off  SenseAxis=off  SenseAngle1=off  SenseAngle2=off  SenseAngle3=off  SenseQ=on  SenseR=off  SenseOmegaX=off  SenseOmegaY=off  SenseOmegaZ=off  SenseOmega1=off  SenseOmega2=off  SenseOmega3=off  SenseQDot=off  SenseRDot=off  SenseAlphaX=off  SenseAlphaY=off  SenseAlphaZ=off  SenseAlpha1=off  SenseAlpha2=off  SenseAlpha3=off  SenseQDDot=off  SenseRDDot=off  SenseX=on  SenseY=on  SenseZ=on  SenseRad=off  SenseAzim=off  SenseDist=off  SenseInc=off  SenseXDot=off  SenseYDot=off  SenseZDot=off  SenseRadDot=off  SenseAzimDot=off  SenseDistDot=off  SenseIncDot=off  SenseXDDot=off  SenseYDDot=off  SenseZDDot=off  SenseRadDDot=off  SenseAzimDDot=off  SenseDistDDot=off  SenseIncDDot=off  BlockFunction=simmechanics.library.frames_transforms.transform_sensor
  World Frame : sm_lib/Frames and Transforms/World Frame  BlockFunction=simmechanics.library.frames_transforms.world_frame
  Frame : PMIOPort  Port=1  Side=Left
  tag scope: QYawShaft=global, xyzYawShaft=global
  wires:
  PS-Simulink Converter/1 -> [QYawShaft]
  PS-Simulink Converter1/1 -> Mux/1
  PS-Simulink Converter2/1 -> Mux/2
  PS-Simulink Converter3/1 -> Mux/3
  Mux/1 -> [xyzYawShaft]
  connections:
  Transform Sensor/RConn1 -- Frame/RConn1
  Transform Sensor/LConn1 -- World Frame/RConn1
  Transform Sensor/RConn3 -- PS-Simulink Converter1/LConn1
  Transform Sensor/RConn4 -- PS-Simulink Converter2/LConn1
  Transform Sensor/RConn5 -- PS-Simulink Converter3/LConn1
  Transform Sensor/RConn2 -- PS-Simulink Converter/LConn1

== system ATRIAS_anim_static_floor/ATRIAS Mechanics Layer/ATRIAS Mechanical System Layer/L Leg/Four Bar Link/Frame Data ==
  Mux : Mux  Inputs=3
  PS-Simulink Converter{,1..3} (4 alike) : nesl_utility/PS-Simulink Converter  PhysicalDomain=network_engine_domain  SubClassName=ps_output  LeftPortType=input  RightPortType=output  PseudoPeriodic=off  Frequencies=[]  Unit=1  AffineConversion=off
  Transform Sensor : sm_lib/Frames and Transforms/Transform Sensor  MeasurementFrame=World  SenseAngle=off  SenseAxis=off  SenseAngle1=off  SenseAngle2=off  SenseAngle3=off  SenseQ=on  SenseR=off  SenseOmegaX=off  SenseOmegaY=off  SenseOmegaZ=off  SenseOmega1=off  SenseOmega2=off  SenseOmega3=off  SenseQDot=off  SenseRDot=off  SenseAlphaX=off  SenseAlphaY=off  SenseAlphaZ=off  SenseAlpha1=off  SenseAlpha2=off  SenseAlpha3=off  SenseQDDot=off  SenseRDDot=off  SenseX=on  SenseY=on  SenseZ=on  SenseRad=off  SenseAzim=off  SenseDist=off  SenseInc=off  SenseXDot=off  SenseYDot=off  SenseZDot=off  SenseRadDot=off  SenseAzimDot=off  SenseDistDot=off  SenseIncDot=off  SenseXDDot=off  SenseYDDot=off  SenseZDDot=off  SenseRadDDot=off  SenseAzimDDot=off  SenseDistDDot=off  SenseIncDDot=off  BlockFunction=simmechanics.library.frames_transforms.transform_sensor
  World Frame : sm_lib/Frames and Transforms/World Frame  BlockFunction=simmechanics.library.frames_transforms.world_frame
  Frame : PMIOPort  Port=1  Side=Left
  tag scope: LQFBlink=global, LxyzFBlink=global
  wires:
  PS-Simulink Converter/1 -> [LQFBlink]
  PS-Simulink Converter1/1 -> Mux/1
  PS-Simulink Converter2/1 -> Mux/2
  PS-Simulink Converter3/1 -> Mux/3
  Mux/1 -> [LxyzFBlink]
  connections:
  Transform Sensor/RConn1 -- Frame/RConn1
  Transform Sensor/LConn1 -- World Frame/RConn1
  Transform Sensor/RConn2 -- PS-Simulink Converter/LConn1
  Transform Sensor/RConn5 -- PS-Simulink Converter3/LConn1
  Transform Sensor/RConn3 -- PS-Simulink Converter1/LConn1
  Transform Sensor/RConn4 -- PS-Simulink Converter2/LConn1

== system ATRIAS_anim_static_floor/ATRIAS Mechanics Layer/ATRIAS Mechanical System Layer/L Leg/Lower Leg/Frame Data ==
  Mux : Mux  Inputs=3
  PS-Simulink Converter{,1..3} (4 alike) : nesl_utility/PS-Simulink Converter  PhysicalDomain=network_engine_domain  SubClassName=ps_output  LeftPortType=input  RightPortType=output  PseudoPeriodic=off  Frequencies=[]  Unit=1  AffineConversion=off
  Transform Sensor : sm_lib/Frames and Transforms/Transform Sensor  MeasurementFrame=World  SenseAngle=off  SenseAxis=off  SenseAngle1=off  SenseAngle2=off  SenseAngle3=off  SenseQ=on  SenseR=off  SenseOmegaX=off  SenseOmegaY=off  SenseOmegaZ=off  SenseOmega1=off  SenseOmega2=off  SenseOmega3=off  SenseQDot=off  SenseRDot=off  SenseAlphaX=off  SenseAlphaY=off  SenseAlphaZ=off  SenseAlpha1=off  SenseAlpha2=off  SenseAlpha3=off  SenseQDDot=off  SenseRDDot=off  SenseX=on  SenseY=on  SenseZ=on  SenseRad=off  SenseAzim=off  SenseDist=off  SenseInc=off  SenseXDot=off  SenseYDot=off  SenseZDot=off  SenseRadDot=off  SenseAzimDot=off  SenseDistDot=off  SenseIncDot=off  SenseXDDot=off  SenseYDDot=off  SenseZDDot=off  SenseRadDDot=off  SenseAzimDDot=off  SenseDistDDot=off  SenseIncDDot=off  BlockFunction=simmechanics.library.frames_transforms.transform_sensor
  World Frame : sm_lib/Frames and Transforms/World Frame  BlockFunction=simmechanics.library.frames_transforms.world_frame
  Frame : PMIOPort  Port=1  Side=Left
  tag scope: LQLowerLeg=global, LxyzLowerLeg=global
  wires:
  PS-Simulink Converter/1 -> [LQLowerLeg]
  PS-Simulink Converter1/1 -> Mux/1
  PS-Simulink Converter2/1 -> Mux/2
  PS-Simulink Converter3/1 -> Mux/3
  Mux/1 -> [LxyzLowerLeg]
  connections:
  Transform Sensor/RConn1 -- Frame/RConn1
  Transform Sensor/LConn1 -- World Frame/RConn1
  Transform Sensor/RConn4 -- PS-Simulink Converter2/LConn1
  Transform Sensor/RConn2 -- PS-Simulink Converter/LConn1
  Transform Sensor/RConn5 -- PS-Simulink Converter3/LConn1
  Transform Sensor/RConn3 -- PS-Simulink Converter1/LConn1

== system ATRIAS_anim_static_floor/ATRIAS Mechanics Layer/ATRIAS Mechanical System Layer/L Leg/Shin/Frame Data ==
  Mux : Mux  Inputs=3
  PS-Simulink Converter{,1..3} (4 alike) : nesl_utility/PS-Simulink Converter  PhysicalDomain=network_engine_domain  SubClassName=ps_output  LeftPortType=input  RightPortType=output  PseudoPeriodic=off  Frequencies=[]  Unit=1  AffineConversion=off
  Transform Sensor : sm_lib/Frames and Transforms/Transform Sensor  MeasurementFrame=World  SenseAngle=off  SenseAxis=off  SenseAngle1=off  SenseAngle2=off  SenseAngle3=off  SenseQ=on  SenseR=off  SenseOmegaX=off  SenseOmegaY=off  SenseOmegaZ=off  SenseOmega1=off  SenseOmega2=off  SenseOmega3=off  SenseQDot=off  SenseRDot=off  SenseAlphaX=off  SenseAlphaY=off  SenseAlphaZ=off  SenseAlpha1=off  SenseAlpha2=off  SenseAlpha3=off  SenseQDDot=off  SenseRDDot=off  SenseX=on  SenseY=on  SenseZ=on  SenseRad=off  SenseAzim=off  SenseDist=off  SenseInc=off  SenseXDot=off  SenseYDot=off  SenseZDot=off  SenseRadDot=off  SenseAzimDot=off  SenseDistDot=off  SenseIncDot=off  SenseXDDot=off  SenseYDDot=off  SenseZDDot=off  SenseRadDDot=off  SenseAzimDDot=off  SenseDistDDot=off  SenseIncDDot=off  BlockFunction=simmechanics.library.frames_transforms.transform_sensor
  World Frame : sm_lib/Frames and Transforms/World Frame  BlockFunction=simmechanics.library.frames_transforms.world_frame
  Frame : PMIOPort  Port=1  Side=Left
  tag scope: LQShin=global, LxyzShin=global
  wires:
  PS-Simulink Converter/1 -> [LQShin]
  PS-Simulink Converter1/1 -> Mux/1
  PS-Simulink Converter2/1 -> Mux/2
  PS-Simulink Converter3/1 -> Mux/3
  Mux/1 -> [LxyzShin]
  connections:
  Transform Sensor/RConn1 -- Frame/RConn1
  Transform Sensor/LConn1 -- World Frame/RConn1
  Transform Sensor/RConn3 -- PS-Simulink Converter1/LConn1
  Transform Sensor/RConn4 -- PS-Simulink Converter2/LConn1
  Transform Sensor/RConn2 -- PS-Simulink Converter/LConn1
  Transform Sensor/RConn5 -- PS-Simulink Converter3/LConn1
